simulink model "fir_fft"  (R2024a)
settings: Solver=VariableStepAuto  StartTime=0.0  StopTime=1024*16  RelTol=1e-3
PreLoadFcn:
  | test_tap32_fft128;
values from neighbouring files (symbols this model uses):
  NUM_OF_FRAMES = 1    [test_tap32_fft128.m]
  taps_td = zeros(1,32)    [test_tap32_fft128.m]
  tmp = double(int16(tmp*2^16))/2^16    [test_tap32_fft128.m]
undefined symbols (not defined in the file or in its folder): None, S, vsva2197, xcvc1902
libraries: aieBasic x5, aieDSP x2, dspobslib x1, vmcUtilities x1
settings Model: Creator=abehbood  LastModifiedBy=robg
settings RTWCC: GPUComputeCapability=3.5
settings ConfigComp: CovBoundaryAbsTol=1.0e-5

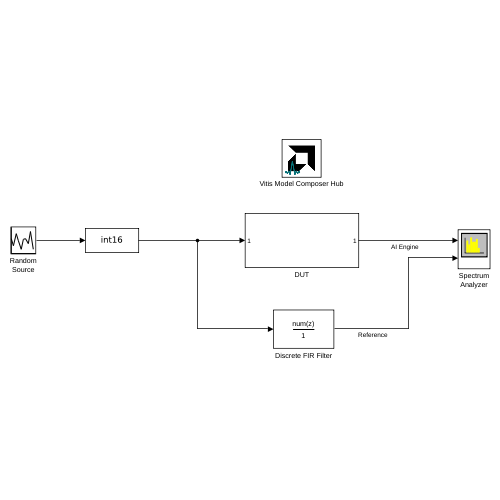
[thumbnail: Simulink's stored preview of the top-level diagram]
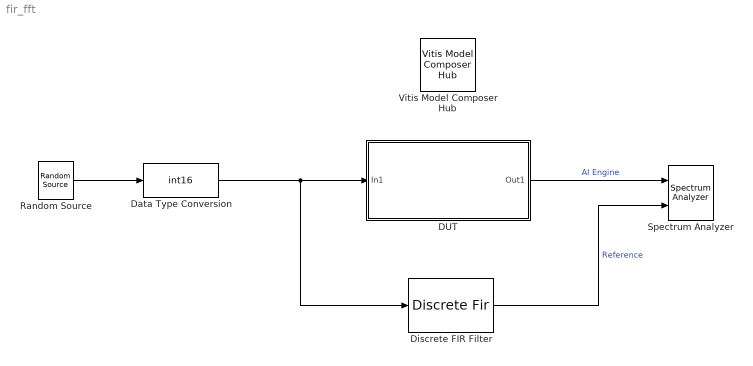
== system fir_fft ==
  DUT : Subsystem
  Data Type Conversion : DataTypeConversion  OutDataTypeStr=int16  SaturateOnIntegerOverflow=off  RndMeth=Floor
  Discrete FIR Filter : DiscreteFir  Coefficients=taps_td  InputProcessing=Columns as channels (frame based)  RndMeth=Convergent  SaturateOnIntegerOverflow=on  OutDataTypeStr=Inherit: Same as input
  Random Source : dspobslib/Random Source  SrcType=Uniform  NormMethod=Ziggurat  CltLength=12  MinVal=-2^8  MaxVal=2^8  MeanVal=0  VarVal=200  RepMode=Not repeatable  rawSeed=1  IsInherit=off  SampMode=Discrete  SampTime=1  SampFrame=96*NUM_OF_FRAMES  DataType=Double  OutComplex=Complex  OutputFrames=off
  Spectrum Analyzer : SpectrumAnalyzer  NumInputPorts=2  WindowPosition=[643.000000,171.000000,880.000000,450.000000,]  ScopeFrameLocation=window  SampleRate=1  Span=1  StartFrequency=-0.5  StopFrequency=0.5  AveragingMethod=Exponential  YLimits=[-6.6857 55.6528]  ShowLegend=on  ChannelNames="[\"\"]"  AllowFFTLengthLessThanSamplesPerUpdate=on  DefaultConfigurationName=spbscopes.SpectrumAnalyzerBlockCfg
  Vitis Model Composer Hub : vmcUtilities/Vitis Model Composer Hub  Tag=genX  CodeGeneration=off  SubsystemName=DUT  BlockHierPath=fir_fft/DUT  SubsystemType=AIENode  AIEArrayConfig=Use entire AIE array  StartColumn=1  NumberOfColumns=1  TargetDirectory=./code  exportDesign=on  analyzeDesign=off  validateDesignOnHw=off  ExportType=HW Code  IpVendor=xilinx.com  IpLibrary=hls  IpVersion=1.0  IpHWLanguage=Verilog  AieCompilerOptions={}  AieSimulatorOptions={}  CreateTestbench=on  TestbenchStackSize=10  RunRtlSim=off  RunCSim=off  RunAieSim=off  AieSimTimeout=50000  RunAieSimProfiling=off  LaunchVitisAnalyzer=off  PlotOutput=off  RunX86Sim=off  X86SimTimeout=10  GenHwImage=off  GenLibadfXo=off  GenHwValidationCode=off  PlatformType=Specify Platform  Platform=/proj/xbuilds/SWIP/9999.0_0722_1852/installs/lin64/2025.2/Vitis/base_platforms/xilinx_vck190_base_202520_1/xilinx_vck190_base_202520_1.xpfm  HwSystemType=Baremetal  HwValidationTarget=hw  ProjDevice=Versal VCK190 Evaluation Platform (xcvc1902-vsva2197-2MP-e-S)  ProjDevicePart=xcvc1902-vsva2197-2MP-e-S  AIEType=AIE  SamplePeriod=-1  ClockFrequency=200  DataPathParallelism=1  xilinxfamily=versalaicore  part=xcvc1902  speed=-2MP-e-S  package=vsva2197  directory=./netlist  testbench=off  incr_netlist=off  synthesis_tool=Vivado  clock_wrapper=Clock Enables  dbl_ovrd=According to Block Masks  dcm_input_clock_period=10  sysclk_period=10  simulink_period=1  eval_field=0  IPInfoJsonString="{\"DUTSubsystemName\":\"DUT\",\"AIESubsystem\":{\"SubsystemName\":\"DUT\",\"TargetDirectory\":\"./code\",\"AIEArrayConfig\":\"Use entire AIE array\",\"StartColumn\":\"0\",\"NumberOfColumns\":\"1\"},\"SubsystemTag\":\"AIENode\"}"  LogFileName=/proj/xhdhdstaff5/sdegala/Head1/HEAD/VMC_JULY_LATEST/Vitis_Model_Composer/Examples/AIENGINE/Filtering_in_frequency_domain/code/model_composer.log  NThreads=4  IPConfigFile=/tmp/vmctmp-12280401783293953895/fir_fft_ipconfig.json
  wires:
  Random Source/1 -> Data Type Conversion/1
  Data Type Conversion/1 -> Discrete FIR Filter/1, DUT/1(In1)
  Discrete FIR Filter/1 -> Spectrum Analyzer/2  "Reference"
  DUT/1(Out1) -> Spectrum Analyzer/1  "AI Engine"

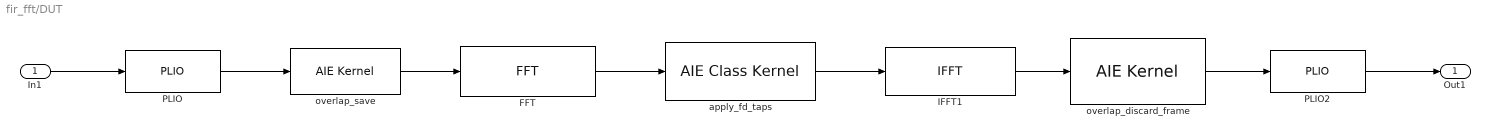
== system fir_fft/DUT ==
  In1 : Inport
  FFT : aieDSP/FFT  AIE_VARIANT=1  data_type=cint16  data_out_type=cint16  twiddle_type=cint16  point_size=128  input_window_size=128*NUM_OF_FRAMES  shift_val=4  rnd_mode=Round symmetrical to infinity  sat_mode=0-None  ssr=1  twiddle_mode=0  use_ssr_widget_kernels=off  casc_length=4  transform_fft_nifft=1  TP_API=0  TP_DYN_PT_SIZE=0  blockJsonConstraints=[]  blockJsonConstraintsInternal=[]  spec=vmc_fft.json  SerializedMaskParamNames=[]  SerializedMaskParamValues=[]  SerializedMaskParamVisibilities=[]  block_type=FFT  SerializedMaskParamDataypes=uint|typename|typename|typename|uint|uint|uint|uint|uint|uint|uint|uint|uint|uint|uint|uint  SerializedMaskParamEnumStrArr=0|0|0|0|0|0|0|Round to positive infinity,Round to negative infinity,Round symmetrical to infinity,Round symmetrical to zero,Round convergent to even,Round convergent to odd|0-None,1-Asymmetric,3-Symmetric|0|0|0|0|0|0|0  SerializedMaskParamEnumValArr=0|0|0|0|0|0|0|2,3,4,5,6,7|0,1,3|0|0|0|0|0|0|0  SerializedMaskParamVectorArr=0|0|0|0|0|0|0|0|0|0|0|0|0|0|0|0  SerializedMaskParamKeys=AIE_VARIANT|TT_DATA|TT_OUT_DATA|TT_TWIDDLE|TP_POINT_SIZE|TP_WINDOW_VSIZE|TP_SHIFT|TP_RND|TP_SAT|TP_PARALLEL_POWER|TP_TWIDDLE_MODE|TP_USE_WIDGETS|TP_CASC_LEN|TP_FFT_NIFFT|TP_API|TP_DYN_PT_SIZE
  IFFT1 : aieDSP/IFFT  data_type=cint16  data_out_type=cint16  twiddle_type=cint16  point_size=128  input_window_size=128*NUM_OF_FRAMES  shift_val=3  rnd_mode=Round symmetrical to infinity  sat_mode=0-None  ssr=1  twiddle_mode=0  use_ssr_widget_kernels=off  casc_length=4  AIE_VARIANT=1  transform_fft_nifft=0  TP_API=0  TP_DYN_PT_SIZE=0  blockJsonConstraints=[]  blockJsonConstraintsInternal=[]  spec=vmc_ifft.json  SerializedMaskParamNames=[]  SerializedMaskParamValues=[]  SerializedMaskParamVisibilities=[]  block_type=IFFT  SerializedMaskParamDataypes=typename|typename|typename|uint|uint|uint|uint|uint|uint|uint|uint|uint|uint|uint|uint|uint  SerializedMaskParamEnumStrArr=0|0|0|0|0|0|Round to positive infinity,Round to negative infinity,Round symmetrical to infinity,Round symmetrical to zero,Round convergent to even,Round convergent to odd|0-None,1-Asymmetric,3-Symmetric|0|0|0|0|0|0|0|0  SerializedMaskParamEnumValArr=0|0|0|0|0|0|2,3,4,5,6,7|0,1,3|0|0|0|0|0|0|0|0  SerializedMaskParamVectorArr=0|0|0|0|0|0|0|0|0|0|0|0|0|0|0|0  SerializedMaskParamKeys=TT_DATA|TT_OUT_DATA|TT_TWIDDLE|TP_POINT_SIZE|TP_WINDOW_VSIZE|TP_SHIFT|TP_RND|TP_SAT|TP_PARALLEL_POWER|TP_TWIDDLE_MODE|TP_USE_WIDGETS|TP_CASC_LEN|AIE_VARIANT|TP_FFT_NIFFT|TP_API|TP_DYN_PT_SIZE
  PLIO : aieBasic/PLIO  PlioWidth=32  PlioFreqSpec=on  PlioFreq=500  ColLocation=0  channel=0  blockJsonConstraints=[]  deprecateConstraints=0
  PLIO2 : aieBasic/PLIO  PlioWidth=32  PlioFreqSpec=on  PlioFreq=500  ColLocation=0  channel=0  blockJsonConstraints=[]  deprecateConstraints=0
  apply_fd_taps : aieBasic/AIE Class Kernel  KernelAllAttrs=|  PortNames={'win_i'; 'win_o'}  PortSerializedTypes={'{Q2{R{Tadf::input_buffer{1{t{Scint16}}}}}}'; '{Q2{R{Tadf::output_buffer{1{t{Scint16}}}}}}'}  PortWindowSizes={1.280000000000000000e+02; 1.280000000000000000e+02}  PortWindowMargins={0.000000000000000000e+00; 0.000000000000000000e+00}  PortSynchronicities={'sync', 'sync'}  PortSignalSizes={0.000000000000000000e+00; 0.000000000000000000e+00}  ClassTemplateSpecKind=implicit  ClassTemplateParamNames={'NUM_OF_FRAMES'}  ClassTemplateParamKinds={'nontype'}  ClassTemplateParamTypes={'int'}  ClassTemplateParamValues={'1'}  ClassCtorParamNames={'taps'}  ClassCtorParamSerializedTypes={'{R{Q1{C{Scint16}128}}}'}  ClassCtorParamValues={'[32767 23173-23173i 0-32767i -23168-23168i -32764 -23169+23169i 0+32767i 23173+23173i 32767 23169-23169i 0-32764i -23170-23170i -32768 -23163+23163i 0+32669i 22924+22924i 31892 21892-21892i 0-29503i -19409-19409i -24795 -15290+15290i 0+18101i 10222+10222i 10937 5497-5497i 0-5137i -2198-2198i -1686 -559+559i 0+299i 54+54i 5 -3+3i 0-2i -3-3i 0 3-3i 0-4i -1-1i 2 2-2i 0-1i 1+1i 4 3-3i 0-1i 2+2i 5 2-2i 0 3+3i 5 3-3i 0 2+2i 5 2-2i 0 2+2i 5 3-3i 0 2+2i 5 2-2i 0 3+3i 5 2-2i 0 2+2i 5 2-2i 0 3+3i 5 3-3i 0 2+2i 5 2-2i 0+1i 3+3i 4 1-1i 0+1i 2+2i 2 -1+1i 0+4i 3+3i 0 -3+3i 0+2i -3-3i 5 54-54i 0-299i -559-559i -1686 -2198+2198i 0+5137i 5497+5497i 10937 10222-10222i 0-18101i -15290-15290i -24795 -19409+19409i 0+29503i 21892+21892i 31892 22924-22924i 0-32669i -23163-23163i -32768 -23170+23170i 0+32764i 23169+23169i 32767 23173-23173i 0-32768i -23169-23169i -32764 -23168+23168i 0+32767i 23173+23173i]'}  ClassIndex=1  ClassCtorIndex=1  ClassTabVisible=on  ClassTemplateParamsVisible=on  ClassCtorDeclVisible=on  ClassCtorParamsVisible=on  FunctionTabVisible=on  FunctionDecl=|  PortAttrs={ 'input', 'win_i', 'adf::input_buffer< cint16 > & restrict', 'NUM_OF_FRAMES*128', '0', 'sync', ''; 'output', 'win_o', 'adf::output_buffer< cint16 > & restrict', 'NUM_OF_FRAMES*128', '', 'sync', '' }  PortAttrsEnables={'off', 'off', 'off', 'on', 'off', 'off', 'off';'off', 'off', 'off', 'on', 'off', 'off', 'off'}  SampleTime=-1  ClassDeclTypeOptions=C[1 1]@t49@template < int NUM_OF_FRAMES > class ApplyFdTaps;  ClassDecl=template < int NUM_OF_FRAMES > class ApplyFdTaps;  ClassTemplateParams={ 'NUM_OF_FRAMES', 'int', 'NUM_OF_FRAMES' }  ClassTemplateParamsEnables={'off', 'off', 'on'}  ClassCtorDeclTypeOptions=C[1 1]@t44@ApplyFdTaps(cint16 const ( & taps ) [ 128 ])  ClassCtorDecl=ApplyFdTaps(cint16 const ( & taps ) [ 128 ])  ClassCtorParams={ 'taps', 'cint16 const ( &) [ 128 ]', 'taps_fd*2^15' }  KernelHeaderFile=kernels/kernels.h  KernelClassName=ApplyFdTaps  KernelFunction=apply_fd_taps  KernelSourceFile=kernels/apply_fd_taps.cpp  KernelSearchPaths={}  PreProcOptions={}  blockJsonConstraints=[]
      KernelAllAttrs=|
      | s[12;12;9;9;19;14;21;23;21;23;24;21;15;17;12;24;26;26;26;27;28;9;21;23;23;23;24;25;14;19;19;29]@FunctionNameDeclFileNamePortNamesPortTypesPortSerializedTypesPortDirectionsPortWindowSizeEnablesPortWindowMarginEnablesPortBufferSizeEnablesPortBufferMarginEnablesPortSynchronicityEnablesPortSignalSizeEnablesPortBufferSizesPortBufferMarginsFunctionDeclFunctionTemplateSpecKindFunctionTemplateParamNamesFunctionTemplateParamKindsFunctionTemplateParamTypesFunctionTemplateParamValuesFunctionTemplateParamEnablesClassDeclClassTemplateSpecKindClassTemplateParamNamesClassTemplateParamKindsClassTemplateParamTypesClassTemplateParamValuesClassTemplateParamEnablesClassCtorDeclsClassCtorParamNamesClassCtorParamTypesClassCtorParamSerializedTypes[1 1]@C[32 1]@t13@apply_fd_tapst23@../../kernels/kernels.hC[2 1]@t5@win_it5@win_oC[2 1]@t38@adf::input_buffer< cint16 > & restrictt39@adf::output_buffer< cint16 > & restrictC[2 1]@t42@{Q2{R{Tadf::input_buffer{1{t{Scint16}}}}}}t43@{Q2{R{Tadf::output_buffer{1{t{Scint16}}}}}}C[2 1]@t5@inputt6@outputC[2 1]@l1@l1@C[2 1]@l1@l0@C[2 1]@l1@l1@C[2 1]@l0@l0@C[2 1]@l1@l1@C[2 1]@l0@l0@C[2 1]@nnC[2 1]@nnt157@template < int NUM_OF_FRAMES > 
      | void ApplyFdTaps::
      | apply_fd_taps(adf::input_buffer< cint16 > & restrict win_i, adf::output_buffer< cint16 > & restrict win_o)t4@nonee[0 1]@e[0 1]@e[0 1]@e[0 1]@e[0 1]@t49@template < int NUM_OF_FRAMES > class ApplyFdTaps;t8@implicitC[1 1]@t13@NUM_OF_FRAMESC[1 1]@t7@nontypeC[1 1]@t3@intC[1 1]@nC[1 1]@l1@C[1 1]@t44@ApplyFdTaps(cint16 const ( & taps ) [ 128 ])C[1 1]@C[1 1]@t4@tapsC[1 1]@C[1 1]@t25@cint16 const ( &) [ 128 ]C[1 1]@C[1 1]@t22@{R{Q1{C{Scint16}128}}}
      FunctionDecl=|
      | template < int NUM_OF_FRAMES > 
      | void ApplyFdTaps::
      | apply_fd_taps(adf::input_buffer< cint16 > & restrict win_i, adf::output_buffer< cint16 > & restrict win_o)
  overlap_discard_frame : aieBasic/AIE Kernel  KernelAllAttrs=|  PortNames={'win_i'; 'win_o'}  PortSerializedTypes={'{Q2{R{Tadf::input_buffer{1{t{Scint16}}}}}}'; '{Q2{R{Tadf::output_buffer{1{t{Scint16}}}}}}'}  PortWindowSizes={1.280000000000000000e+02, 9.600000000000000000e+01}  PortWindowMargins={0.000000000000000000e+00, 0.000000000000000000e+00}  PortSynchronicities={'sync', 'sync'}  PortSignalSizes={0.000000000000000000e+00; 0.000000000000000000e+00}  FunctionTemplateSpecKind=implicit  FunctionTemplateParamNames={'NUM_OF_FRAMES'}  FunctionTemplateParamKinds={'nontype'}  FunctionTemplateParamTypes={'int'}  FunctionTemplateParamValues={'1'}  FunctionIndex=1  FunctionTabVisible=on  FunctionTemplateParamsVisible=on  FunctionDeclTypeOptions=|  FunctionDecl=|  FunctionTemplateParams={ 'NUM_OF_FRAMES', 'int', 'NUM_OF_FRAMES' }  FunctionTemplateParamsEnables={'off', 'off', 'on'}  PortAttrs={ 'input', 'win_i', 'adf::input_buffer< cint16 > & restrict', 'NUM_OF_FRAMES*128', '0', 'sync', ''; 'output', 'win_o', 'adf::output_buffer< cint16 > & restrict', 'NUM_OF_FRAMES*96', '', 'sync', '' }  PortAttrsEnables={'off', 'off', 'off', 'on', 'off', 'off', 'off';'off', 'off', 'off', 'on', 'off', 'off', 'off'}  SampleTime=-1  KernelHeaderFile=kernels/kernels.h  KernelFunction=overlap_discard  KernelSourceFile=kernels/overlap_discard.cpp  KernelSearchPaths={}  PreProcOptions={}  blockJsonConstraints=[]
      KernelAllAttrs=|
      | s[12;12;9;9;19;14;21;23;21;23;24;21;15;17;12;24;26;26;26;27;28;9;21;23;23;23;24;25;14;19;19;29]@FunctionNameDeclFileNamePortNamesPortTypesPortSerializedTypesPortDirectionsPortWindowSizeEnablesPortWindowMarginEnablesPortBufferSizeEnablesPortBufferMarginEnablesPortSynchronicityEnablesPortSignalSizeEnablesPortBufferSizesPortBufferMarginsFunctionDeclFunctionTemplateSpecKindFunctionTemplateParamNamesFunctionTemplateParamKindsFunctionTemplateParamTypesFunctionTemplateParamValuesFunctionTemplateParamEnablesClassDeclClassTemplateSpecKindClassTemplateParamNamesClassTemplateParamKindsClassTemplateParamTypesClassTemplateParamValuesClassTemplateParamEnablesClassCtorDeclsClassCtorParamNamesClassCtorParamTypesClassCtorParamSerializedTypes[1 1]@C[32 1]@t15@overlap_discardt23@../../kernels/kernels.hC[2 1]@t5@win_it5@win_oC[2 1]@t38@adf::input_buffer< cint16 > & restrictt39@adf::output_buffer< cint16 > & restrictC[2 1]@t42@{Q2{R{Tadf::input_buffer{1{t{Scint16}}}}}}t43@{Q2{R{Tadf::output_buffer{1{t{Scint16}}}}}}C[2 1]@t5@inputt6@outputC[2 1]@l1@l1@C[2 1]@l1@l0@C[2 1]@l1@l1@C[2 1]@l0@l0@C[2 1]@l1@l1@C[2 1]@l0@l0@C[2 1]@nnC[2 1]@nnt145@template < int NUM_OF_FRAMES > 
      | void overlap_discard(adf::input_buffer< cint16 > & restrict win_i, adf::output_buffer< cint16 > & restrict win_o)t8@implicitC[1 1]@t13@NUM_OF_FRAMESC[1 1]@t7@nontypeC[1 1]@t3@intC[1 1]@nC[1 1]@l1@nne[0 1]@e[0 1]@e[0 1]@e[0 1]@e[0 1]@e[0 1]@e[0 1]@e[0 1]@e[0 1]@
      FunctionDeclTypeOptions=|
      | C[1 1]@t147@template < int NUM_OF_FRAMES > 
      | void overlap_discard(adf::input_buffer< cint16 > && restrict win_i, adf::output_buffer< cint16 > && restrict win_o)
      FunctionDecl=|
      | template < int NUM_OF_FRAMES > 
      | void overlap_discard(adf::input_buffer< cint16 > && restrict win_i, adf::output_buffer< cint16 > && restrict win_o)
  overlap_save : aieBasic/AIE Kernel  KernelAllAttrs=|  PortNames={'win_i'; 'win_o'}  PortSerializedTypes={'{Q2{R{Tadf::input_buffer{3{t{Scint16}}{t{Tadf::extents{1{t{}adf::inherited_extent}}}}{t{Tadf::margin{1{t{}32}}}}}}}}'; '{Q2{R{Tadf::output_buffer{1{t{Scint16}}}}}}'}  PortWindowSizes={9.600000000000000000e+01, 1.280000000000000000e+02}  PortWindowMargins={3.200000000000000000e+01, 0.000000000000000000e+00}  PortSynchronicities={'sync', 'sync'}  PortSignalSizes={0.000000000000000000e+00; 0.000000000000000000e+00}  FunctionTemplateSpecKind=implicit  FunctionTemplateParamNames={'NUM_OF_FRAMES'}  FunctionTemplateParamKinds={'nontype'}  FunctionTemplateParamTypes={'int'}  FunctionTemplateParamValues={'1'}  FunctionIndex=1  FunctionTabVisible=on  FunctionTemplateParamsVisible=on  FunctionDeclTypeOptions=|  FunctionDecl=|  FunctionTemplateParams={ 'NUM_OF_FRAMES', 'int', 'NUM_OF_FRAMES' }  FunctionTemplateParamsEnables={'off', 'off', 'on'}  PortAttrs={ 'input', 'win_i', 'adf::input_buffer< cint16, adf::extents< adf::inherited_extent >, adf::margin< 32 > > & restrict', 'NUM_OF_FRAMES*96', '32', 'sync', ''; 'output', 'win_o', 'adf::output_buffer< cint16 > & restrict', 'NUM_OF_FRAMES*128', '', 'sync', '' }  PortAttrsEnables={'off', 'off', 'off', 'on', 'off', 'off', 'off';'off', 'off', 'off', 'on', 'off', 'off', 'off'}  SampleTime=-1  KernelHeaderFile=kernels/kernels.h  KernelFunction=overlap_save  KernelSourceFile=kernels/overlap_save.cpp  KernelSearchPaths={}  PreProcOptions={}  blockJsonConstraints=[]
      KernelAllAttrs=|
      | s[12;12;9;9;19;14;21;23;21;23;24;21;15;17;12;24;26;26;26;27;28;9;21;23;23;23;24;25;14;19;19;29]@FunctionNameDeclFileNamePortNamesPortTypesPortSerializedTypesPortDirectionsPortWindowSizeEnablesPortWindowMarginEnablesPortBufferSizeEnablesPortBufferMarginEnablesPortSynchronicityEnablesPortSignalSizeEnablesPortBufferSizesPortBufferMarginsFunctionDeclFunctionTemplateSpecKindFunctionTemplateParamNamesFunctionTemplateParamKindsFunctionTemplateParamTypesFunctionTemplateParamValuesFunctionTemplateParamEnablesClassDeclClassTemplateSpecKindClassTemplateParamNamesClassTemplateParamKindsClassTemplateParamTypesClassTemplateParamValuesClassTemplateParamEnablesClassCtorDeclsClassCtorParamNamesClassCtorParamTypesClassCtorParamSerializedTypes[1 1]@C[32 1]@t12@overlap_savet23@../../kernels/kernels.hC[2 1]@t5@win_it5@win_oC[2 1]@t96@adf::input_buffer< cint16, adf::extents< adf::inherited_extent >, adf::margin< 32 > > & restrictt39@adf::output_buffer< cint16 > & restrictC[2 1]@t116@{Q2{R{Tadf::input_buffer{3{t{Scint16}}{t{Tadf::extents{1{t{}adf::inherited_extent}}}}{t{Tadf::margin{1{t{}32}}}}}}}}t43@{Q2{R{Tadf::output_buffer{1{t{Scint16}}}}}}C[2 1]@t5@inputt6@outputC[2 1]@l1@l1@C[2 1]@l1@l0@C[2 1]@l1@l1@C[2 1]@l0@l0@C[2 1]@l1@l1@C[2 1]@l0@l0@C[2 1]@nnC[2 1]@t2@32nt200@template < int NUM_OF_FRAMES > 
      | void overlap_save(adf::input_buffer< cint16, adf::extents< adf::inherited_extent >, adf::margin< 32 > > & restrict win_i, adf::output_buffer< cint16 > & restrict win_o)t8@implicitC[1 1]@t13@NUM_OF_FRAMESC[1 1]@t7@nontypeC[1 1]@t3@intC[1 1]@nC[1 1]@l1@nne[0 1]@e[0 1]@e[0 1]@e[0 1]@e[0 1]@e[0 1]@e[0 1]@e[0 1]@e[0 1]@
      FunctionDeclTypeOptions=|
      | C[1 1]@t202@template < int NUM_OF_FRAMES > 
      | void overlap_save(adf::input_buffer< cint16, adf::extents< adf::inherited_extent >, adf::margin< 32 > > && restrict win_i, adf::output_buffer< cint16 > && restrict win_o)
      FunctionDecl=|
      | template < int NUM_OF_FRAMES > 
      | void overlap_save(adf::input_buffer< cint16, adf::extents< adf::inherited_extent >, adf::margin< 32 > > && restrict win_i, adf::output_buffer< cint16 > && restrict win_o)
  Out1 : Outport
  wires:
  In1/1 -> PLIO/1
  PLIO/1 -> overlap_save/1
  overlap_discard_frame/1 -> PLIO2/1
  PLIO2/1 -> Out1/1
  overlap_save/1 -> FFT/1
  FFT/1 -> apply_fd_taps/1
  IFFT1/1 -> overlap_discard_frame/1
  apply_fd_taps/1 -> IFFT1/1
